simulink model "TP09_Ej10"  (R2020b)
settings: Solver=FixedStepAuto  StartTime=0.0  StopTime=10  FixedStep=1e-3  RelTol=1e-3  EnableMultiTasking=on
settings Model: Creator=54115  LastModifiedBy=Juan
settings DataIOCC: ReturnWorkspaceOutputs=off
settings OptimizationCC: LifeSpan=inf
settings DebuggingCC: SFUnexpectedBacktrackingDiag=warning  SFNoUnconditionalDefaultTransitionDiag=warning  ArithmeticOperatorsInVariantConditions=warning
settings SFSimCC: SimUseLocalCustomCode=off  CustomCodeUndefinedFunction=UseInterfaceOnly
settings RTWCC: RTWUseLocalCustomCode=off
settings CodeAppCC: StateflowObjectComments=on
settings GRTTargetCC: TargetLangStandard=C89/C90 (ANSI)
settings ConfigComp: CovMetricSettings=dw  CovSaveCumulativeToWorkspaceVar=on  CovSaveSingleToWorkspaceVar=on  CovExternalEMLEnable=off

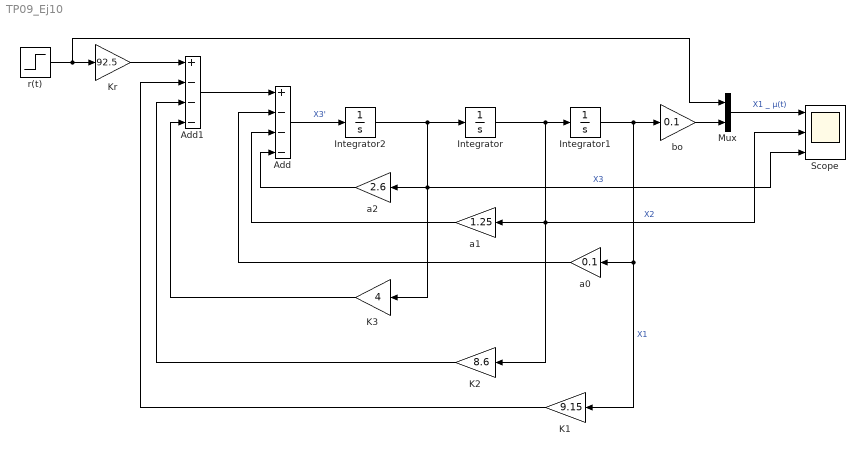
== system TP09_Ej10 ==
  Add : Sum  Inputs=+---
  Add1 : Sum  Inputs=+---
  Integrator : Integrator
  Integrator1 : Integrator
  Integrator2 : Integrator
  K1 : Gain  Gain=9.15
  K2 : Gain  Gain=8.6
  K3 : Gain  Gain=4
  Kr : Gain  Gain=92.5
  Mux : Mux  Inputs=2
  Scope : Scope  NumInputPorts=3
  a0 : Gain  Gain=0.1
  a1 : Gain  Gain=1.25
  a2 : Gain  Gain=2.6
  bo : Gain  Gain=0.1
  r(t) : Step  Time=0  SampleTime=0
  wires:
  Integrator2/1 -> Integrator/1, Scope/3, K3/1, a2/1  "X3"
  Integrator/1 -> Scope/2, K2/1, a1/1, Integrator1/1  "X2"
  Add/1 -> Integrator2/1  "X3'"
  a2/1 -> Add/4
  a1/1 -> Add/3
  Integrator1/1 -> bo/1, K1/1, a0/1  "X1"
  Mux/1 -> Scope/1  "X1 _ μ(t)"
  Add1/1 -> Add/1
  r(t)/1 -> Kr/1, Mux/1
  K3/1 -> Add1/4
  K2/1 -> Add1/3
  a0/1 -> Add/2
  K1/1 -> Add1/2
  bo/1 -> Mux/2
  Kr/1 -> Add1/1
